simulink model "exsim3modelPart1"  (R2018b)
settings: Solver=VariableStepAuto  StartTime=0.0  StopTime=10.0  RelTol=1e-3
values from neighbouring files (symbols this model uses):
  Kc = 2    [exsim3.m]
  Ts = 0.2    [exsim3.m]
libraries: simulink x1
settings Model: Creator=rafael  LastModifiedBy=rafael

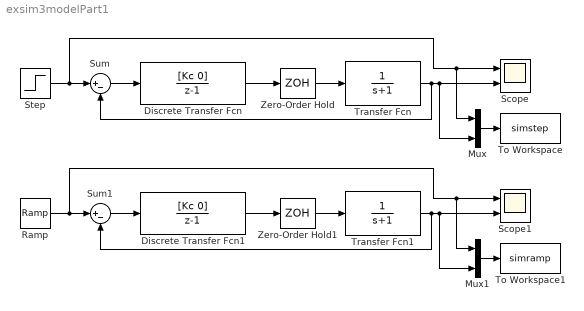
== system exsim3modelPart1 ==
  Discrete Transfer Fcn : DiscreteTransferFcn  Numerator=[Kc 0]  Denominator=[1 -1]  SampleTime=Ts
  Discrete Transfer Fcn1 : DiscreteTransferFcn  Numerator=[Kc 0]  Denominator=[1 -1]  SampleTime=Ts
  Mux : Mux  Inputs=2
  Mux1 : Mux  Inputs=2
  Ramp : simulink/Sources/Ramp  slope=1  start=0  InitialOutput=0
  Scope : Scope  NumInputPorts=2
  Scope1 : Scope  NumInputPorts=2
  Step : Step  SampleTime=0
  Sum : Sum  Inputs=|+-
  Sum1 : Sum  Inputs=|+-
  To Workspace : ToWorkspace  VariableName=simstep  SaveFormat=Timeseries  SampleTime=-1
  To Workspace1 : ToWorkspace  VariableName=simramp  SaveFormat=Timeseries  SampleTime=-1
  Transfer Fcn : TransferFcn  Denominator=[1 1]
  Transfer Fcn1 : TransferFcn  Denominator=[1 1]
  Zero-Order Hold : ZeroOrderHold  SampleTime=Ts
  Zero-Order Hold1 : ZeroOrderHold  SampleTime=Ts
  wires:
  Step/1 -> Mux/1, Scope/1, Sum/1
  Sum/1 -> Discrete Transfer Fcn/1
  Zero-Order Hold/1 -> Transfer Fcn/1
  Transfer Fcn/1 -> Mux/2, Scope/2, Sum/2
  Discrete Transfer Fcn/1 -> Zero-Order Hold/1
  Mux/1 -> To Workspace/1
  Discrete Transfer Fcn1/1 -> Zero-Order Hold1/1
  Transfer Fcn1/1 -> Mux1/2, Scope1/2, Sum1/2
  Mux1/1 -> To Workspace1/1
  Sum1/1 -> Discrete Transfer Fcn1/1
  Zero-Order Hold1/1 -> Transfer Fcn1/1
  Ramp/1 -> Mux1/1, Scope1/1, Sum1/1
